simulink model "TD3_simu"  (R2017b)
settings: Solver=VariableStepAuto  StartTime=0.0  StopTime=4.0  RelTol=1e-3
values from neighbouring files (symbols this model uses):
  Cr = 0    [MCC_variables.m]    (also in TD3.m)
  J = 3.2284e-6    (= 3.2284e-06)    [MCC_variables.m]    (also in TD2_config.m = 0.28; TD3.m = 0.2)
  Lo = 12.16e-3    (= 0.01216)    [TD3.m]
  p = 3    [TD3.m]
  phi = K/p    (= 0.3)    [TD3.m]
  psi = pi/4    (= 0.785398163397)    [TD3.m]
  R = 4    [MCC_variables.m]    (also in TD2_config.m = 0.015; TD3.m = 0.895)
  Uo = 220    [TD3.m]
settings Model: Creator=Table2  LastModifiedBy=Table2

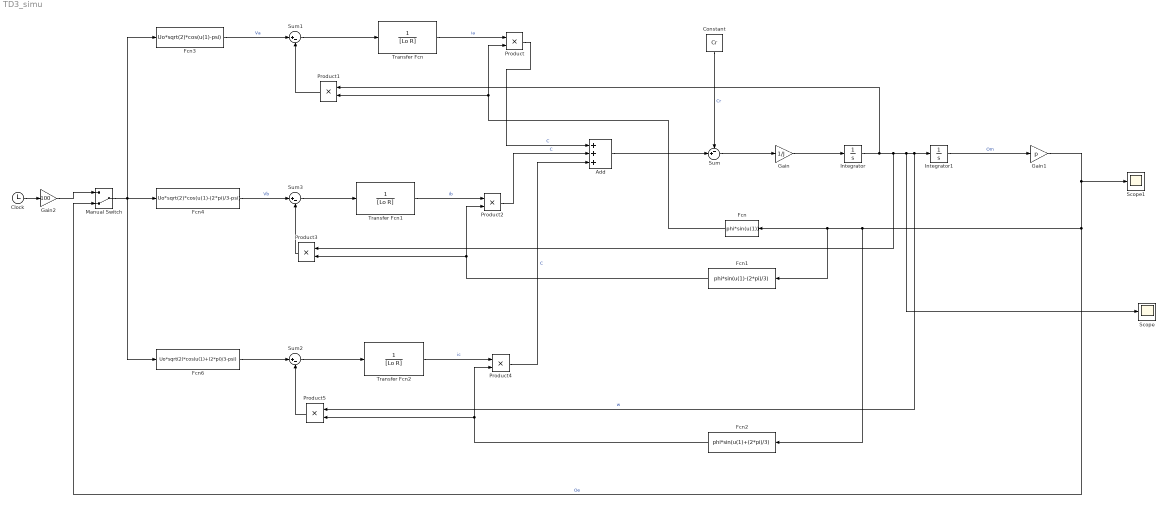
== system TD3_simu ==
  Add : Sum  Inputs=+++
  Clock : Clock
      settings: Decimation=4
  Constant : Constant  Value=Cr
  Fcn : Fcn  Expr=phi*sin(u(1))
  Fcn1 : Fcn  Expr=phi*sin(u(1)-(2*pi)/3)
  Fcn2 : Fcn  Expr=phi*sin(u(1)+(2*pi)/3)
  Fcn3 : Fcn  Expr=Uo*sqrt(2)*cos(u(1)-psi)
  Fcn4 : Fcn  Expr=Uo*sqrt(2)*cos(u(1)-(2*pi)/3-psi)
  Fcn6 : Fcn  Expr=Uo*sqrt(2)*cos(u(1)+(2*pi)/3-psi)
  Gain : Gain  Gain=1/J
  Gain1 : Gain  Gain=p
  Gain2 : Gain  Gain=100
  Integrator : Integrator
  Integrator1 : Integrator
  Manual Switch : ManualSwitch  CurrentSetting=0
  Product{,1..5} (6 alike) : Product
  Scope : Scope
  Scope1 : Scope
  Sum : Sum  Inputs=-+|
  Sum1 : Sum  Inputs=|+-
  Sum2 : Sum  Inputs=|+-
  Sum3 : Sum  Inputs=|+-
  Transfer Fcn : TransferFcn  Denominator=[Lo R]
  Transfer Fcn1 : TransferFcn  Denominator=[Lo R]
  Transfer Fcn2 : TransferFcn  Denominator=[Lo R]
  wires:
  Fcn3/1 -> Sum1/1  "Va"
  Sum1/1 -> Transfer Fcn/1
  Transfer Fcn/1 -> Product/1  "ia"
  Constant/1 -> Sum/1  "Cr"
  Sum/1 -> Gain/1
  Gain/1 -> Integrator/1
  Integrator1/1 -> Gain1/1  "Om"
  Fcn/1 -> Product1/2, Product/2
  Product1/1 -> Sum1/2
  Sum3/1 -> Transfer Fcn1/1
  Transfer Fcn1/1 -> Product2/1  "ib"
  Fcn4/1 -> Sum3/1  "Vb"
  Product3/1 -> Sum3/2
  Fcn1/1 -> Product3/2, Product2/2
  Add/1 -> Sum/2
  Product/1 -> Add/1  "C"
  Product2/1 -> Add/2  "C"
  Product4/1 -> Add/3  "C"
  Transfer Fcn2/1 -> Product4/1  "ic"
  Fcn2/1 -> Product5/2, Product4/2
  Product5/1 -> Sum2/2
  Gain1/1 -> Scope1/1, Manual Switch/2, Fcn2/1, Fcn1/1, Fcn/1  "Oe"
  Integrator/1 -> Product1/1, Product3/1, Scope/1, Product5/1, Integrator1/1  "w"
  Sum2/1 -> Transfer Fcn2/1
  Fcn6/1 -> Sum2/1
  Clock/1 -> Gain2/1
  Manual Switch/1 -> Fcn6/1, Fcn3/1, Fcn4/1
  Gain2/1 -> Manual Switch/1
